simulink model "motor"  (R2017b)
settings: Solver=VariableStepAuto  StartTime=0.0  StopTime=1  RelTol=1e-3
values from neighbouring files (symbols this model uses):
  dd = [1 -1.864 .8694]    [control.m]
  kp = 30    [control.m]
  nd = [0 .0008826 0]    [control.m]
  T0 = 0.005    [control.m]
undefined symbols (not defined in the file or in its folder): DiscIntNeverNeededParam
libraries: simulink x1
settings Model: Creator=Agustin  LastModifiedBy=Agustin

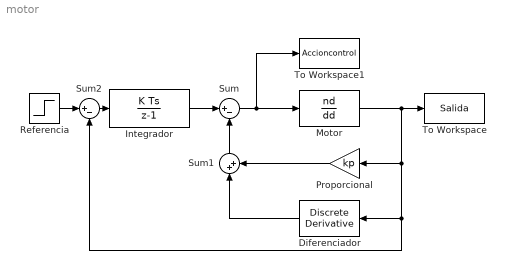
== system motor ==
  Diferenciador : simulink/Discrete/Discrete Derivative  gainval=kd  ICPrevScaledInput=0.0  OutMin=[]  OutMax=[]  OutDataType=fixdt(1, 16)  OutScaling=2^-10  DoSatur=off
  Integrador : DiscreteIntegrator  gainval=ki  InitialConditionSetting=State (most efficient)  SampleTime=T0  ICPrevOutput=DiscIntNeverNeededParam  ICPrevScaledInput=DiscIntNeverNeededParam
  Motor : DiscreteTransferFcn  Numerator=nd  Denominator=dd  SampleTime=T0
  Proporcional : Gain  Gain=kp
  Referencia : Step  Time=0  After=1.5  SampleTime=T0
  Sum : Sum  Inputs=|+-
  Sum1 : Sum  Inputs=|++
  Sum2 : Sum  Inputs=|+-
  To Workspace : ToWorkspace  VariableName=Salida  SaveFormat=Timeseries  SampleTime=-1
  To Workspace1 : ToWorkspace  VariableName=Accioncontrol  SaveFormat=Timeseries  SampleTime=-1
  wires:
  Motor/1 -> Sum2/2, Diferenciador/1, Proporcional/1, To Workspace/1
  Integrador/1 -> Sum/1
  Diferenciador/1 -> Sum1/1
  Proporcional/1 -> Sum1/2
  Sum1/1 -> Sum/2
  Sum2/1 -> Integrador/1
  Referencia/1 -> Sum2/1
  Sum/1 -> To Workspace1/1, Motor/1
